simulink model "Estimation_model_4P_GSUAUCI"  (R2018b)
settings: Solver=ode4  StartTime=0.0  StopTime=265  FixedStep=0.01  MaxStep=0.01  RelTol=1e-3  EnableMultiTasking=on
model workspace (MAT data in the model file):
  A_c1 = 1
  A_c2 = -0.75
  A_c3 = -0.75
  A_c4 = 1
  C = 220000
  Delta_tc1 = 6.5
  Delta_tc2 = 6.5
  Delta_tc3 = 6.5
  Delta_tc4 = 6.5
  E0 = 15000
  He0 = 50
  Hi0 = 8
  Hr0 = 0
  Hs0 = 275000
  L0 = 15000
  Me0 = 650
  Mi0 = 50
  Ms0 = 5005000
  P0 = 15000
  alfa = 1.3
  alpha = 1.3
  beta_h = 2
  beta_m = 2
  delta = 100
  dt_c1 = 6.5
  dt_c2 = 6.5
  dt_c3 = 6.5
  dt_c4 = 6.5
  f = 0.5
  gamma_e = 1.15
  gamma_h = 1.15
  gamma_l = 0.8
  gamma_p = 0.85
  mu_e = 0.65
  mu_h = 0.000455
  mu_l = 1.61
  mu_m = 0.45
  mu_p = 0.7
  t0_c1 = 34
  t0_c2 = 127
  t0_c3 = 225
  t0_c4 = 250
  theta_h = 1.1
  theta_m = 0.7
settings Model: Creator=MATERO  LastModifiedBy=alex
settings DataIOCC: SaveFormat=Array  SignalLogging=off  DSMLogging=off  ReturnWorkspaceOutputs=on  SignalLoggingName=Hi  OutputTimes=tout  ReturnWorkspaceOutputsName=SDOSimTest_Log
settings OptimizationCC: LifeSpan=inf
settings DebuggingCC: UnderspecifiedInitializationDetection=Classic  MergeDetectMultiDrivingBlocksExec=none  MaxConsecutiveZCsMsg=warning  SolverPrmCheckMsg=warning  ModelReferenceExtraNoncontSigs=warning  StateNameClashWarn=warning  SFUnexpectedBacktrackingDiag=warning  SFNoUnconditionalDefaultTransitionDiag=warning  SFExecutionAtInitializationDiag=none
settings HardwareCC: ProdBitPerPointer=32  ProdBitPerSizeT=32  ProdBitPerPtrDiffT=32  ProdLargestAtomicFloat=None  ProdIntDivRoundTo=Undefined  ProdEndianess=Unspecified  ProdWordSize=32  ProdHWDeviceType=32-bit Generic
settings ModelReferenceCC: PropagateSignalLabelsOutOfModel=off
settings SFSimCC: SimUseLocalCustomCode=off
settings RTWCC: RTWUseLocalCustomCode=off
settings CodeAppCC: StateflowObjectComments=on
settings GRTTargetCC: TargetLangStandard=C89/C90 (ANSI)  GeneratePreprocessorConditionals=Disable all
settings ConfigComp: CovMetricSettings=dw  CovHtmlReporting=on  CovSaveCumulativeToWorkspaceVar=on  CovSaveSingleToWorkspaceVar=on  CovExternalEMLEnable=off

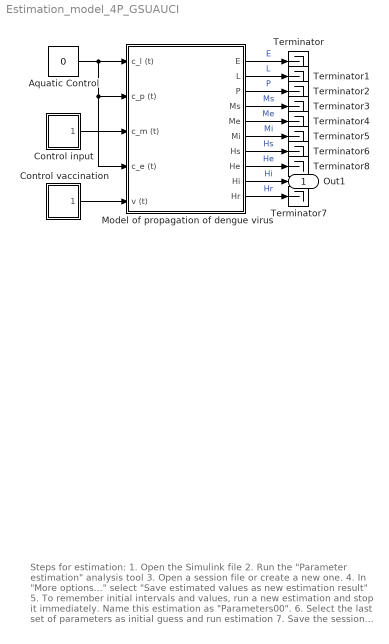
== system Estimation_model_4P_GSUAUCI ==
  note: Steps for estimation:
      | 1. Open the Simulink file
      | 2. Run the "Parameter estimation" analysis tool
      | 3. Open a session file or create a new one.
      | 4. In "More options..." select "Save estimated values
      | as new estimation result"
      | 5. To remember initial intervals and values, run a new
      | estimation and stop it immediately. Name this estimation
      | as "Parameters00".
      | 6. Select the last set of parameters as initial guess and run estimation
      | 7. Save the session as a file "Estimation xx (explanation)"
      | 8. Run the script "Results_SDOInfo.m" to see the results and save
      | them to Excel sheet "Test" in file "SDOInfoExcel.xlsx"
  Aquatic Control : Constant  Value=0
  Control input : Subsystem  mask(Continuous-time pulse){A_c1=A_c1, t0_c1=t0_c1, dt_c1=dt_c1, A_c2=A_c2, t0_c2=t0_c2, dt_c2=dt_c2, A_c3=A_c3, t0_c3=t0_c3, dt_c3=dt_c3, A_c4=A_c4, t0_c4=t0_c4, dt_c4=dt_c4}
      mask prompts: A_c1 "Amplitude 1"; t0_c1 "Initial time 1"; dt_c1 "Pulse width (time) 1"; A_c2 "Amplitude 2"; t0_c2 "Initial time 2"; dt_c2 "Pulse width (time) 2"; A_c3 "Amplitude 3"; t0_c3 "Initial time 3"; dt_c3 "pulse width (time) 3"; A_c4 "Amplitude 4"; t0_c4 "Initial time 4"; dt_c4 "pulse width (time) 4"
      mask init:
      | t0_c1=round(t0_c1,2);
      | t0_c2=round(t0_c2,2);
      | t0_c3=round(t0_c3,2);
      | t0_c4=round(t0_c4,2);
      | 
      | dt_c1=round(dt_c1,2);
      | dt_c2=round(dt_c2,2);
      | dt_c3=round(dt_c3,2);
      | dt_c4=round(dt_c4,2);
      | 
      | wp_1 = dt_c1*100/1e6;
      | wp_2 = dt_c2*100/1e6;
      | wp_3 = dt_c3*100/1e6;
      | wp_4 = dt_c4*100/1e6;
      mask Display: plot([0 0.4 0.4 0.8 0.8 1.2],[0 0 0.8 0.8 0 0])
  Control vaccination : Subsystem  mask(Continuous-time pulse){v=0, t0_v=1, dt_v=1}
      mask prompts: v "Amplitude 1"; t0_v "Initial time 1"; dt_v "Pulse width (time) 1"
      mask init:
      | t0_v=round(t0_v,2);
      | 
      | dt_v=round(dt_v,2);
      | 
      | wp_1 = dt_v*100/1e6;
      mask Display: plot([0 0.4 0.4 0.8 0.8 1.2],[0 0 0.8 0.8 0 0])
  Model of propagation of dengue virus : Subsystem  mask(Modelo EAFIT de propagación del dengue){ciA=[E0, L0, P0], ciM=[Ms0 Me0 Mi0], ciH=[Hs0 He0 Hi0 Hr0], delta=delta, C=C, gamma_e=gamma_e, mu_e=mu_e, gamma_l=gamma_l, mu_l=mu_l, gamma_p=gamma_p, mu_p=mu_p, f=f, beta_m=beta_m, mu_m=mu_m, theta_m=theta_m, mu_h=mu_h, beta_h=beta_h, theta_h=theta_h, gamma_h=gamma_h, v=0, alfa=alpha}
      mask prompts: ciA "Condiciones iniciales de la fase acuática [E0, L0, P0]"; ciM "Condiciones iniciales mosquitos [Ms0, Me0, Mi0]"; ciH "Condiciones iniciales humanos [Hs0, He0, Hi0, Hr0]"; delta "Tasa promedio de oviposición [delta]"; C "Capacidad de carga de los huevos [C]"; gamma_e "Tasa de transición de huevo a larva [gamma_e]"; mu_e "Tasa de mortalidad de huevos [mu_e]"; gamma_l "Tasa de transición de larva a pupa [gamma_l]"; mu_l "Tasa de mortalidad de larvas [mu_l]"; gamma_p "Tasa de transición de pupa a mosquito [gamma_p]"; mu_p "Tasa de mortalidad de pupas [mu_p]"; f "Proporción de mosquitos hembras [f]"; beta_m "Tasa total de transmisión de humano a mosquito [beta_m]"; mu_m "Tasa de mortalidad de mosquitos [mu_m]"; theta_m "Tasa de incubación extrínseca [theta_m]"; mu_h "Tasa de mortalidad humanos [mu_h]"; beta_h "Tasa total de transmisión de mosquito a humano [beta_h]"; theta_h "Tasa de incubación intrínseca [theta_h]"; gamma_h "Tasa de recuperación [gamma_h]"; v "Inmunidad de la poblacion [v]"; alfa "Cambio de mortalidad en Me-Mi"
      mask help:
      | Modelo de 10 estados (E, L, P, Ms, Me, Mi, Hs, He, Hi, Hr) y
      | 5 entradas (eliminación de huevos c_e, eliminación de larvas c_l,
      | eliminación de pupas c_p, fumigación c_m, vacunación c_v)
      mask init:
      | Hs0=ciH(1); He0=ciH(2); Hi0=ciH(3); Hr0=ciH(4);
      | Ms0=ciM(1); Me0=ciM(2); Mi0=ciM(3);
      | E0=ciA(1); L0=ciA(2); P0=ciA(3);
  Terminator{,1..8} (9 alike) : Terminator
  Out1 : Outport
  wires:
  Model of propagation of dengue virus/1("E ") -> Terminator/1  "E"
  Model of propagation of dengue virus/2("L ") -> Terminator1/1  "L"
  Model of propagation of dengue virus/3("P ") -> Terminator2/1  "P"
  Model of propagation of dengue virus/4("Ms ") -> Terminator3/1  "Ms"
  Model of propagation of dengue virus/5("Me ") -> Terminator4/1  "Me"
  Model of propagation of dengue virus/6("Mi ") -> Terminator5/1  "Mi"
  Model of propagation of dengue virus/7("Hs ") -> Terminator6/1  "Hs"
  Model of propagation of dengue virus/8("He ") -> Terminator8/1  "He"
  Model of propagation of dengue virus/9("Hi ") -> Out1/1  "Hi"
  Model of propagation of dengue virus/10(Hr) -> Terminator7/1  "Hr"
  Aquatic Control/1 -> Model of propagation of dengue virus/4(c_e (t)), Model of propagation of dengue virus/2(c_p (t)), Model of propagation of dengue virus/1(c_l (t))
  Control input/1(Out1) -> Model of propagation of dengue virus/3(c_m (t))
  Control vaccination/1(Out1) -> Model of propagation of dengue virus/5(v (t))

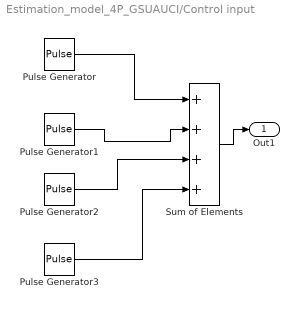
== system Estimation_model_4P_GSUAUCI/Control input ==
  Pulse Generator : DiscretePulseGenerator  PulseType=Time based  Amplitude=A_c1  Period=1e6  PulseWidth=wp_1  PhaseDelay=t0_c1
  Pulse Generator1 : DiscretePulseGenerator  PulseType=Time based  Amplitude=A_c2  Period=1e6  PulseWidth=wp_2  PhaseDelay=t0_c2
  Pulse Generator2 : DiscretePulseGenerator  PulseType=Time based  Amplitude=A_c3  Period=1e6  PulseWidth=wp_3  PhaseDelay=t0_c3
  Pulse Generator3 : DiscretePulseGenerator  PulseType=Time based  Amplitude=A_c4  Period=1e6  PulseWidth=wp_4  PhaseDelay=t0_c4
  Sum of Elements : Sum  Inputs=++++
  Out1 : Outport
  wires:
  Pulse Generator/1 -> Sum of Elements/1
  Pulse Generator1/1 -> Sum of Elements/2
  Sum of Elements/1 -> Out1/1
  Pulse Generator2/1 -> Sum of Elements/3
  Pulse Generator3/1 -> Sum of Elements/4

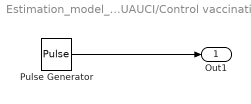
== system Estimation_model_4P_GSUAUCI/Control vaccination ==
  Pulse Generator : DiscretePulseGenerator  PulseType=Time based  Amplitude=v  Period=1e6  PulseWidth=wp_1  PhaseDelay=t0_v
  Out1 : Outport
  wires:
  Pulse Generator/1 -> Out1/1

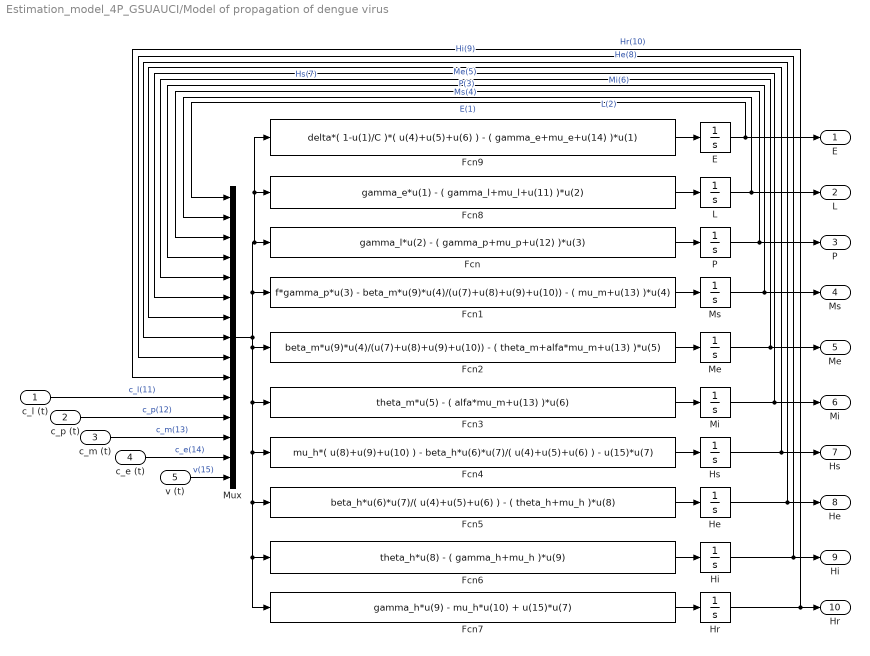
== system Estimation_model_4P_GSUAUCI/Model of propagation of dengue virus ==
  c_l (t) : Inport
  c_p (t) : Inport  Port=2
  c_m (t) : Inport  Port=3
  c_e (t) : Inport  Port=4
  v (t) : Inport  Port=5
  E : Integrator  InitialCondition=E0  LimitOutput=on  LowerSaturationLimit=0
  Fcn : Fcn  Expr=gamma_l*u(2) - ( gamma_p+mu_p+u(12) )*u(3)
  Fcn1 : Fcn  Expr="f*gamma_p*u(3)  - beta_m*u(9)*u(4)/(u(7)+u(8)+u(9)+u(10))  - ( mu_m+u(13) )*u(4)"
  Fcn2 : Fcn  Expr=beta_m*u(9)*u(4)/(u(7)+u(8)+u(9)+u(10)) - ( theta_m+alfa*mu_m+u(13) )*u(5)
  Fcn3 : Fcn  Expr=theta_m*u(5) - ( alfa*mu_m+u(13) )*u(6)
  Fcn4 : Fcn  Expr=mu_h*( u(8)+u(9)+u(10) ) - beta_h*u(6)*u(7)/( u(4)+u(5)+u(6) ) - u(15)*u(7)
  Fcn5 : Fcn  Expr=beta_h*u(6)*u(7)/( u(4)+u(5)+u(6) ) - ( theta_h+mu_h )*u(8)
  Fcn6 : Fcn  Expr=theta_h*u(8) - ( gamma_h+mu_h )*u(9)
  Fcn7 : Fcn  Expr=gamma_h*u(9) - mu_h*u(10) + u(15)*u(7)
  Fcn8 : Fcn  Expr=gamma_e*u(1) - ( gamma_l+mu_l+u(11) )*u(2)
  Fcn9 : Fcn  Expr=delta*( 1-u(1)/C )*( u(4)+u(5)+u(6) ) - ( gamma_e+mu_e+u(14) )*u(1)
  He : Integrator  InitialCondition=He0  LimitOutput=on  LowerSaturationLimit=0
  Hi : Integrator  InitialCondition=Hi0  LimitOutput=on  LowerSaturationLimit=0
  "Hr " : Integrator  InitialCondition=Hr0  LimitOutput=on  LowerSaturationLimit=0
  Hs : Integrator  InitialCondition=Hs0  LimitOutput=on  LowerSaturationLimit=0
  L : Integrator  InitialCondition=L0  LimitOutput=on  LowerSaturationLimit=0
  Me : Integrator  InitialCondition=Me0  LimitOutput=on  LowerSaturationLimit=0
  Mi : Integrator  InitialCondition=Mi0  LimitOutput=on  LowerSaturationLimit=0
  Ms : Integrator  InitialCondition=Ms0  LimitOutput=on  LowerSaturationLimit=0
  Mux : Mux  Inputs=15
  P : Integrator  InitialCondition=P0  LimitOutput=on  LowerSaturationLimit=0
  "E " : Outport
  "L " : Outport  Port=2
  "P " : Outport  Port=3
  "Ms " : Outport  Port=4
  "Me " : Outport  Port=5
  "Mi " : Outport  Port=6
  "Hs " : Outport  Port=7
  "He " : Outport  Port=8
  "Hi " : Outport  Port=9
  Hr : Outport  Port=10
  wires:
  Fcn/1 -> P/1
  P/1 -> Mux/3, "P "/1  "P(3)"
  Ms/1 -> "Ms "/1, Mux/4  "Ms(4)"
  Me/1 -> Mux/5, "Me "/1  "Me(5)"
  Mi/1 -> "Mi "/1, Mux/6  "Mi(6)"
  Hi/1 -> Mux/9, "Hi "/1  "Hi(9)"
  He/1 -> Mux/8, "He "/1  "He(8)"
  Hs/1 -> Mux/7, "Hs "/1  "Hs(7)"
  Fcn1/1 -> Ms/1
  Fcn2/1 -> Me/1
  Fcn3/1 -> Mi/1
  Fcn4/1 -> Hs/1
  Mux/1 -> Fcn7/1, Fcn6/1, Fcn5/1, Fcn4/1, Fcn3/1, Fcn2/1, Fcn1/1, Fcn9/1, Fcn8/1, Fcn/1
  Fcn5/1 -> He/1
  Fcn6/1 -> Hi/1
  Fcn7/1 -> "Hr "/1
  "Hr "/1 -> Mux/10, Hr/1  "Hr(10)"
  Fcn8/1 -> L/1
  Fcn9/1 -> E/1
  E/1 -> Mux/1, "E "/1  "E(1)"
  L/1 -> "L "/1, Mux/2  "L(2)"
  c_l (t)/1 -> Mux/11  "c_l(11)"
  c_p (t)/1 -> Mux/12  "c_p(12)"
  c_m (t)/1 -> Mux/13  "c_m(13)"
  c_e (t)/1 -> Mux/14  "c_e(14)"
  v (t)/1 -> Mux/15  "v(15)"
